simulink model "servoLower"  (R2022b)
settings: Solver=VariableStepAuto  StartTime=0.0  StopTime=3.0  RelTol=1e-8
settings Model: Creator=HP  LastModifiedBy=HP
settings SolverCC: AlgebraicLoopSolver=TrustRegion
settings DebuggingCC: UnconnectedInputMsg=warning  UnconnectedOutputMsg=warning  UnconnectedLineMsg=warning  SFMachineParentedDataDiag=warning
settings ModelReferenceCC: EnableRefExpFcnMdlSchedulingChecks=on
settings RTWCC: DLArmComputeVersion=19.05

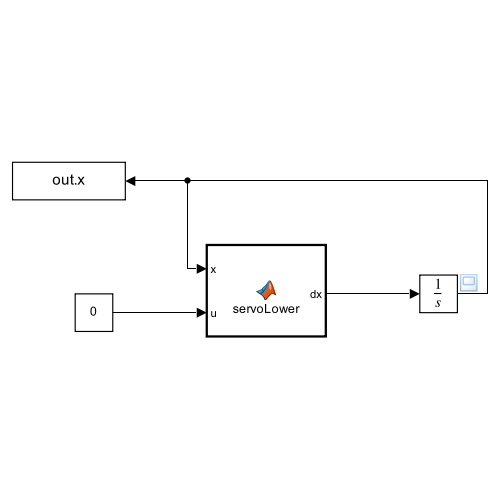
[thumbnail: Simulink's stored preview of the top-level diagram]
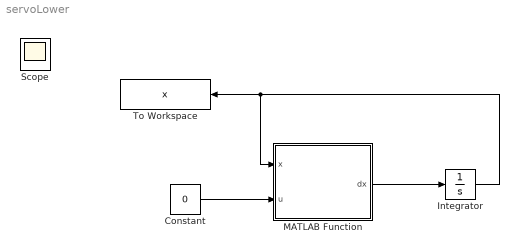
== system servoLower ==
  Constant : Constant  Value=0
  Integrator : Integrator  InitialCondition=[0; pi/8; 0; 0]  IgnoreLimit=on
  MATLAB Function : MATLAB Function  TreatAsAtomicUnit=on
  To Workspace : ToWorkspace  VariableName=x  SaveFormat=Timeseries  SampleTime=-1
  Scope : Scope
  wires:
  MATLAB Function/1(dx) -> Integrator/1
  Integrator/1 -> MATLAB Function/1(x), To Workspace/1
  Constant/1 -> MATLAB Function/2(u)

== matlab function servoLower/MATLAB Function ==
  data: x input; u input; dx output
function dx = servoLower(x, u)
ltefunction dx = servoLower(x,u)
%% Motor
% Resistance
Rm = 8.4;
% Current-torque (N-m/A)
kt = 0.042;
% Back-emf constant (V-s/rad)
km = 0.042;
%
%% Rotary Arm
% Mass (kg)
mr = 0.095;
% Total length (m)
r = 0.085;
% Moment of inertia about pivot (kg-m^2)
Jr = mr*r^2/3;
% Equivalent Viscous Damping Coefficient (N-m-s/rad)
br = 1e-3; % damping tuned heuristically to match QUBE-Sero 2 response
%
%% Pendulum Link
% Mass (kg)
mp = 0.024;
% Total length (m)
Lp = 0.129;
% Pendulum center of mass (m)
l = Lp/2;
% Moment of inertia about pivot (kg-m^2)
Jp = mp*Lp^2/3;
% Equivalent Viscous Damping Coefficient (N-m-s/rad)
bp = 5e-5; % damping tuned heuristically to match QUBE-Sero 2 response
% Gravity Constant
g = 9.81;
Jt=Jp*Jr-mp^2*l^2*r^2;
%Control voltage and the torque
%%
% state vectors 

%%
%matrix forms 
A=[ 0   0                      1                         0;
    0   0                      0                         1;
    0, g*l^2*mp^2*r/Jt,     -(Jp*br)/Jt,               bp*l*mp*r/Jt;
    0, -Jr*g*l*mp/Jt,           br*l*mp*r/Jt,              -Jr*bp /Jt];
 

B=[0; 0; Jp/Jt; -mp*r*l/Jt];
C=[1 0 0 0;
   0 1 0 0];
D=[0 ; 0];
dx=A*x+B*u;
